simulink model "data_analysis"  (R2026a)
settings: Solver=FixedStepDiscrete  StopTime=inf  FixedStep=0.001
model workspace (MAT data in the model file):
  RxTree : serdes.internal.ibisami.ami.SerDesTree (value not decoded)
libraries: instrumentseriallib x2
settings Model: Creator=POND  LastModifiedBy=POND

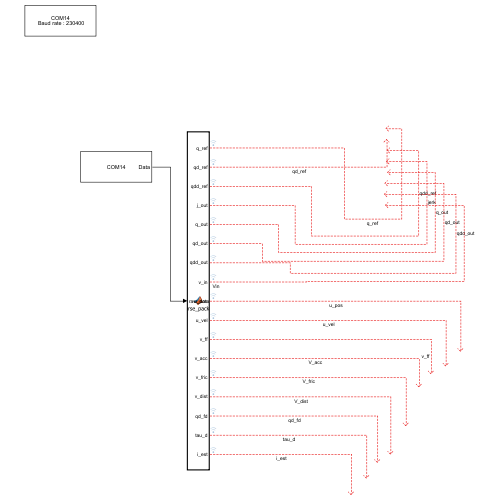
[thumbnail: Simulink's stored preview of the top-level diagram]
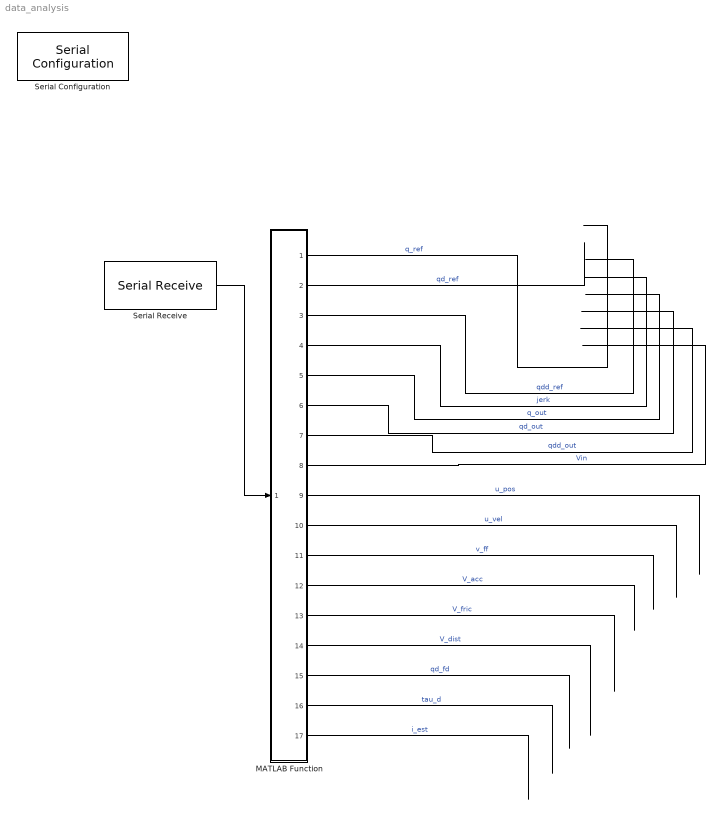
== system data_analysis ==
  MATLAB Function : MATLAB Function  TreatAsAtomicUnit=on
  Serial Configuration : instrumentseriallib/Serial Configuration  Priority=-200000  PortSel=COM14  Port=COM14  ComPort=COM14  BaudRate=230400  DataBits=8  Parity=even  StopBits=1  ByteOrder=little-endian  FlowControl=none  Timeout=0.1  SimulateUsing=Interpreted execution  BlockInModel=on  aMode=1
  Serial Receive : instrumentseriallib/Serial Receive  Priority=1  PortSel=COM14  Port=COM14  ComPort=COM14  DataType=uint8  SaveDataType=uint8  ToggleHeader=on  Header=[170 85]  ToggleDataSize=on  DataSize=[34 1]  ToggleTerminator=off  Terminator=<none>  CustomTerminator=[]  InputFormat=Column major  EnableBlockingMode=on  ActionDataUnavailable=Output last received value  ActionWhenDataUnavailable=Output last received value  CustomValue=0  SampleTime=0.001  SimulateUsing=Interpreted execution  BlockInModel=on  aMode=1  LibraryInUse=instrumentlib
  wires:
  Serial Receive/1 -> MATLAB Function/1(raw_data)
  MATLAB Function/1(q_ref) -> ?  "q_ref"
  MATLAB Function/2(qd_ref) -> ?  "qd_ref"
  MATLAB Function/3(qdd_ref) -> ?  "qdd_ref"
  MATLAB Function/4(j_out) -> ?  "jerk"
  MATLAB Function/5(q_out) -> ?  "q_out"
  MATLAB Function/6(qd_out) -> ?  "qd_out"
  MATLAB Function/7(qdd_out) -> ?  "qdd_out"
  MATLAB Function/8(v_in) -> ?  "Vin"
  MATLAB Function/9(u_pos) -> ?  "u_pos"
  MATLAB Function/10(u_vel) -> ?  "u_vel"
  MATLAB Function/11(v_ff) -> ?  "v_ff"
  MATLAB Function/12(v_acc) -> ?  "V_acc"
  MATLAB Function/13(v_fric) -> ?  "V_fric"
  MATLAB Function/14(v_dist) -> ?  "V_dist"
  MATLAB Function/15(qd_fd) -> ?  "qd_fd"
  MATLAB Function/16(tau_d) -> ?  "tau_d"
  MATLAB Function/17(i_est) -> ?  "i_est"

== matlab function data_analysis/MATLAB Function ==
  data: raw_data input; q_ref output; qd_ref output; qdd_ref output; j_out output; q_out output; qd_out output; qdd_out output; v_in output; u_pos output; u_vel output; v_ff output; v_acc output; v_fric output; v_dist output; qd_fd output; tau_d output; i_est output
function [q_ref, qd_ref, qdd_ref, j_out, q_out, qd_out, qdd_out, v_in, ...
          u_pos, u_vel, v_ff, v_acc, v_fric, v_dist, ...
          qd_fd, tau_d, i_est] = parse_packet(raw_data)
    %#codegen
    persistent last_v;
    if isempty(last_v)
        last_v = zeros(17, 1);
    end

    % Header ถูกตัดโดย Serial Receive block แล้ว → raw_data = payload 34 byte
    if length(raw_data) == 34
        d = typecast(uint8(raw_data(:)'), 'int16');   % 17 × int16 (Little-Endian)

        last_v(1)  = double(d(1))  / 1000.0; % q_ref
        last_v(2)  = double(d(2))  / 1000.0; % qd_ref
        last_v(3)  = double(d(3))  / 100.0;  % qdd_ref
        last_v(4)  = double(d(4))  / 10.0;   % jerk (mon_j_out)
        last_v(5)  = double(d(5))  / 1000.0; % q_out (KF)
        last_v(6)  = double(d(6))  / 1000.0; % qd_out (KF)
        last_v(7)  = double(d(7))  / 100.0;  % qdd_out
        last_v(8)  = double(d(8))  / 1000.0; % v_in
        last_v(9)  = double(d(9))  / 1000.0; % u_pos
        last_v(10) = double(d(10)) / 1000.0; % u_vel
        last_v(11) = double(d(11)) / 1000.0; % v_ff
        last_v(12) = double(d(12)) / 1000.0; % v_acc
        last_v(13) = double(d(13)) / 1000.0; % v_fric
        last_v(14) = double(d(14)) / 1000.0; % v_dist
        last_v(15) = double(d(15)) / 1000.0; % qd_fd
        last_v(16) = double(d(16)) / 1000.0; % tau_d
        last_v(17) = double(d(17)) / 1000.0; % i_est
    end

    q_ref=last_v(1);  qd_ref=last_v(2);  qdd_ref=last_v(3); j_out=last_v(4);
    q_out=last_v(5);  qd_out=last_v(6);  qdd_out=last_v(7); v_in=last_v(8);
    u_pos=last_v(9);  u_vel=last_v(10);  v_ff=last_v(11);   v_acc=last_v(12);
    v_fric=last_v(13);v_dist=last_v(14); qd_fd=last_v(15);  tau_d=last_v(16);
    i_est=last_v(17);
end
